simulink model "system_model"  (R2024b)
settings: Solver=ode4  StartTime=0.0  StopTime=T_stop  FixedStep=0.1  RelTol=1e-3
undefined symbols (not defined in the file): bms, dt, SoC_init, T_cool_init, V_RC1_init, V_RC2_init
libraries: simulink x2
settings Model: DataDictionary=buses.sldd  SimulationMode=accelerator  Creator=rayen  LastModifiedBy=rayen
settings OptimizationCC: ZeroExternalMemoryAtStartup=off  ZeroInternalMemoryAtStartup=off
settings DebuggingCC: AlgebraicLoopMsg=error
settings SFSimCC: SimTargetLang=C++
settings RTWCC: TargetLang=C++
settings GRTTargetCC: TargetLangStandard=C++11 (ISO)  CodeInterfacePackaging=C++ class

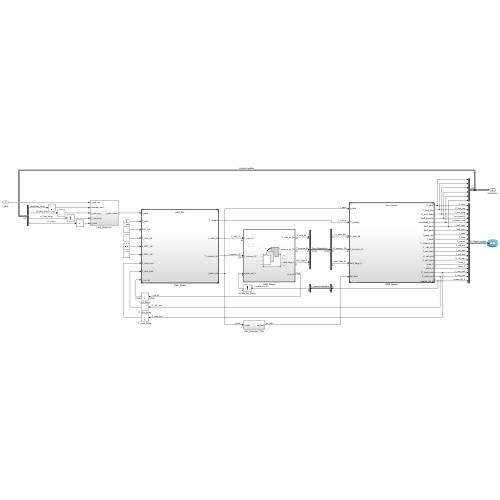
[thumbnail: Simulink's stored preview of the top-level diagram]
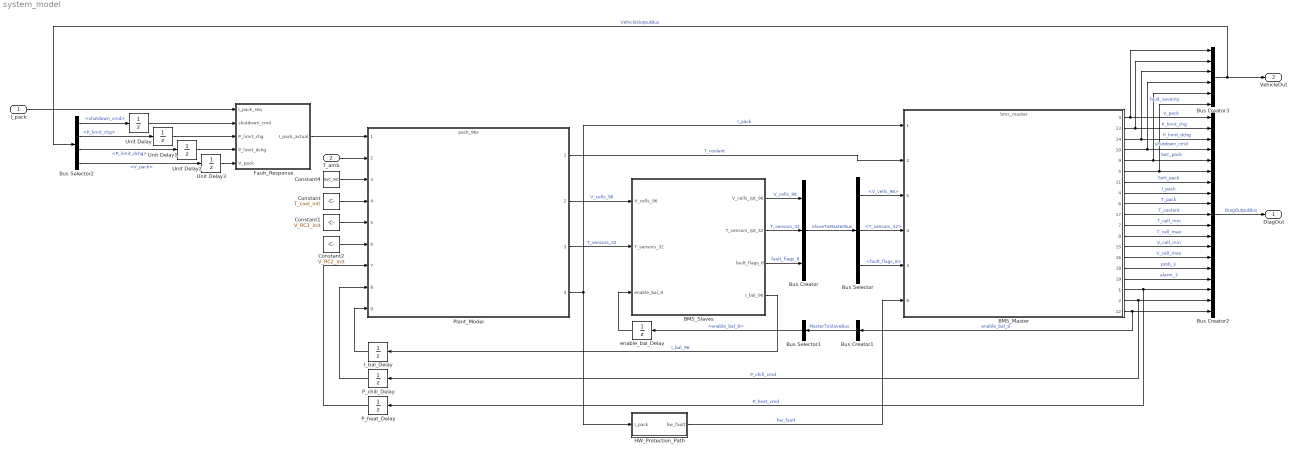
== system system_model ==
  I_pack : Inport  OutDataTypeStr=double
  T_amb : Inport  Port=2  OutDataTypeStr=double
  BMS_Master : ModelReference  ModelNameDialog=bms_master  SimulationMode=Normal  ModelReferenceVersion=1.251
      settings: PortSchema="{\"entries\":[{\"content\":{\"sides\":[{\"content\":{\"connectorIds\":[\"In1\",\"In2\",\"In5\",\"In4\",\"In3\",\"In6\"]},\"type\":\"ConnectorPlacement.EquallySpacedRectSide\",\"uuid\":\"8066489d-2b28-420f-9202-9cd6ff178a29\"},{\"content\":{\"connectorIds\":[\"Out3\",\"Out13\",\"Out14\",\"Out10\",\"Out9\",\"Out5\",\"Out11\",\"Out4\",\"Out6\",\"Out17\",\"Out7\",\"Out8\",\"Out15\",\"Out16\",\"Out18\",\"Out19\",\"Out1\",\"Out2\",\"Out12\"],\"side\":\"RIGHT\"},\"type\":\"ConnectorPlacement.EquallySpacedRectSide\",\"uuid\":\"b076ecb5-2558-4b32-94db-f7a524b49e8a\"},{\"content\":{\"side\":\"TOP\"},\"type\":\"ConnectorPlacement.EquallySpacedRectSide\",\"uuid\":\"5bce71a0-8ae7-4a96-a6b6-c7adac2010e7\"}]},\"type\":\"ConnectorPlacement.EquallySpacedConnector\",\"uuid\":\"27e9bc73-c1a9-451e-b2df-2718d4e67b4c\"}],\"packageUris\":[\"http://schema.mathworks.com/mf0/Connector/R2020b\"],\"version\":\"1.0\"}"
  BMS_Slaves : Subsystem  TreatAsAtomicUnit=on
  Bus Creator : BusCreator  Inputs=3  OutDataTypeStr=Bus: SlaveToMasterBus
  Bus Creator1 : BusCreator  Inputs=1  OutDataTypeStr=Bus: MasterToSlaveBus
  Bus Creator2 : BusCreator  Inputs=19  OutDataTypeStr=Bus: DiagOutputBus
  Bus Creator3 : BusCreator  Inputs=6  OutDataTypeStr=Bus: VehicleOutputBus
  Bus Selector : BusSelector  OutputSignals=V_cells_96,T_sensors_32,fault_flags_8
  Bus Selector1 : BusSelector  OutputSignals=enable_bal_8
  Bus Selector2 : BusSelector  OutputSignals=shutdown_cmd,P_limit_chg,P_limit_dchg,V_pack
  Constant : Constant  Value=T_cool_init
  Constant1 : Constant  Value=V_RC1_init
  Constant2 : Constant  Value=V_RC2_init
  Constant4 : Constant  Value=SoC_init
  Fault_Response : Subsystem
  HW_Protection_Path : Subsystem
  I_bal_Delay : UnitDelay  InitialCondition=zeros(12,8)  SampleTime=dt  HasFrameUpgradeWarning=on
  P_chill_Delay : UnitDelay  SampleTime=dt  HasFrameUpgradeWarning=on
  P_heat_Delay : UnitDelay  SampleTime=dt  HasFrameUpgradeWarning=on
  Plant_Model : ModelReference  ModelNameDialog=pack_96s.slx  SimulationMode=Normal  ModelReferenceVersion=1.65
  Unit Delay : UnitDelay  SampleTime=dt  HasFrameUpgradeWarning=on
  Unit Delay1 : UnitDelay  InitialCondition=96*4.2*150  SampleTime=dt  HasFrameUpgradeWarning=on
  Unit Delay2 : UnitDelay  InitialCondition=96*2.5*405  SampleTime=dt  HasFrameUpgradeWarning=on
  Unit Delay3 : UnitDelay  InitialCondition=96*3.7  SampleTime=dt  HasFrameUpgradeWarning=on
  enable_bal_Delay : UnitDelay  InitialCondition=zeros(1,8)  SampleTime=dt  HasFrameUpgradeWarning=on
  DiagOut : Outport  OutDataTypeStr=Bus: DiagOutputBus
  VehicleOut : Outport  Port=2  OutDataTypeStr=Bus: VehicleOutputBus
  wires:
  T_amb/1 -> Plant_Model/2
  Constant/1 -> Plant_Model/4
  Constant2/1 -> Plant_Model/6
  Constant4/1 -> Plant_Model/3
  Constant1/1 -> Plant_Model/5
  P_heat_Delay/1 -> Plant_Model/7
  Plant_Model/1 -> BMS_Master/2  "T_coolant"
  enable_bal_Delay/1 -> BMS_Slaves/3(enable_bal_8)
  BMS_Slaves/4(I_bal_96) -> I_bal_Delay/1  "I_bal_96"
  I_bal_Delay/1 -> Plant_Model/9
  P_chill_Delay/1 -> Plant_Model/8
  BMS_Slaves/3(fault_flags_8) -> Bus Creator/3  "fault_flags_8"
  BMS_Slaves/2(T_sensors_rpt_32) -> Bus Creator/2  "T_sensors_32"
  BMS_Slaves/1(V_cells_rpt_96) -> Bus Creator/1  "V_cells_96"
  Bus Creator/1 -> Bus Selector/1  "SlaveToMasterBus"
  Bus Creator1/1 -> Bus Selector1/1  "MasterToSlaveBus"
  Bus Selector1/1 -> enable_bal_Delay/1  "<enable_bal_8>"
  Fault_Response/1(I_pack_actual) -> Plant_Model/1
  I_pack/1 -> Fault_Response/1(I_pack_req)
  Unit Delay2/1 -> Fault_Response/4(P_limit_dchg)
  Bus Selector2/2 -> Unit Delay1/1  "<P_limit_chg>"
  Unit Delay3/1 -> Fault_Response/5(V_pack)
  Bus Selector2/4 -> Unit Delay3/1  "<V_pack>"
  Unit Delay1/1 -> Fault_Response/3(P_limit_chg)
  Unit Delay/1 -> Fault_Response/2(shutdown_cmd)
  Bus Selector2/1 -> Unit Delay/1  "<shutdown_cmd>"
  Bus Selector2/3 -> Unit Delay2/1  "<P_limit_dchg>"
  Plant_Model/4 -> HW_Protection_Path/1(I_pack), BMS_Master/1  "I_pack"
  Plant_Model/2 -> BMS_Slaves/1(V_cells_96)  "V_cells_96"
  Plant_Model/3 -> BMS_Slaves/2(T_sensors_32)  "T_sensors_32"
  BMS_Master/3 -> Bus Creator3/1, Bus Creator2/1  "V_pack"
  BMS_Master/13 -> Bus Creator3/2, Bus Creator2/2  "P_limit_chg"
  BMS_Master/14 -> Bus Creator3/3, Bus Creator2/3  "P_limit_dchg"
  BMS_Master/10 -> Bus Creator3/4, Bus Creator2/4  "fault_severity"
  BMS_Master/9 -> Bus Creator3/5, Bus Creator2/5  "shutdown_cmd"
  BMS_Master/5 -> Bus Creator3/6, Bus Creator2/6  "SoC_pack"
  BMS_Master/11 -> Bus Creator2/7  "SoH_pack"
  BMS_Master/4 -> Bus Creator2/8  "I_pack"
  BMS_Master/6 -> Bus Creator2/9  "T_pack"
  BMS_Master/17 -> Bus Creator2/10  "T_coolant"
  BMS_Master/7 -> Bus Creator2/11  "T_cell_min"
  BMS_Master/8 -> Bus Creator2/12  "T_cell_max"
  BMS_Master/15 -> Bus Creator2/13  "V_cell_min"
  BMS_Master/16 -> Bus Creator2/14  "V_cell_max"
  Bus Creator2/1 -> DiagOut/1  "DiagOutputBus"
  Bus Creator3/1 -> VehicleOut/1, Bus Selector2/1  "VehicleOutputBus"
  Bus Selector/1 -> BMS_Master/5  "<V_cells_96>"
  Bus Selector/2 -> BMS_Master/4  "<T_sensors_32>"
  Bus Selector/3 -> BMS_Master/3  "<fault_flags_8>"
  BMS_Master/18 -> Bus Creator2/15  "prob_3"
  BMS_Master/19 -> Bus Creator2/16  "alarm_3"
  BMS_Master/1 -> Bus Creator2/17, P_heat_Delay/1  "P_heat_cmd"
  BMS_Master/2 -> Bus Creator2/18, P_chill_Delay/1  "P_chill_cmd"
  BMS_Master/12 -> Bus Creator1/1, Bus Creator2/19  "enable_bal_8"
  HW_Protection_Path/1(hw_fault) -> BMS_Master/6  "hw_fault"

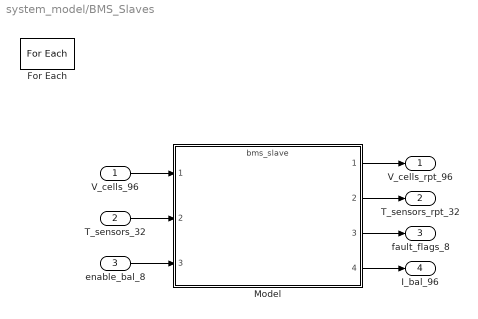
== system system_model/BMS_Slaves ==
  V_cells_96 : Inport  Partition=on  PartitionDimension=1  PartitionWidth=12  PartitionOffset=0
  T_sensors_32 : Inport  Port=2  Partition=on  PartitionDimension=1  PartitionWidth=4  PartitionOffset=0
  enable_bal_8 : Inport  Port=3  Partition=on  PartitionDimension=1  PartitionWidth=1  PartitionOffset=0
  For Each : ForEach  DisableCoverage=on
  Model : ModelReference  ModelNameDialog=bms_slave.slx  ModelReferenceVersion=1.60
  V_cells_rpt_96 : Outport  ConcatenationDimension=1
  T_sensors_rpt_32 : Outport  Port=2  ConcatenationDimension=1
  fault_flags_8 : Outport  Port=3  ConcatenationDimension=1
  I_bal_96 : Outport  Port=4  ConcatenationDimension=2
  wires:
  V_cells_96/1 -> Model/1
  T_sensors_32/1 -> Model/2
  enable_bal_8/1 -> Model/3
  Model/1 -> V_cells_rpt_96/1
  Model/2 -> T_sensors_rpt_32/1
  Model/3 -> fault_flags_8/1
  Model/4 -> I_bal_96/1

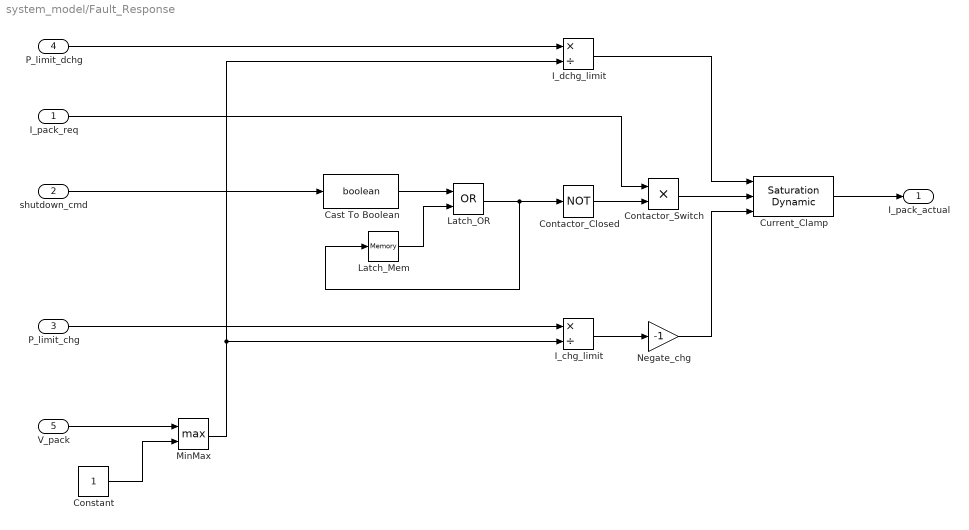
== system system_model/Fault_Response ==
  I_pack_req : Inport
  shutdown_cmd : Inport  Port=2
  P_limit_chg : Inport  Port=3
  P_limit_dchg : Inport  Port=4
  V_pack : Inport  Port=5
  Cast To Boolean : DataTypeConversion  OutDataTypeStr=boolean  SaturateOnIntegerOverflow=off  RndMeth=Floor
  Constant : Constant
  Contactor_Closed : Logic  Operator=NOT  AllPortsSameDT=off  OutDataTypeStr=boolean
  Contactor_Switch : Product
  Current_Clamp : simulink/Discontinuities/Saturation Dynamic  OutMin=[]  OutMax=[]  OutDataTypeStr=Inherit: Same as second input  OutDataType=fixdt(1, 16)  OutScaling=2^-10  DoSatur=off
  I_chg_limit : Product  Inputs=*/
  I_dchg_limit : Product  Inputs=*/
  Latch_Mem : Memory
  Latch_OR : Logic  Operator=OR  AllPortsSameDT=off  OutDataTypeStr=boolean
  MinMax : MinMax  Function=max  Inputs=2
  Negate_chg : Gain  Gain=-1
  I_pack_actual : Outport
  wires:
  Latch_Mem/1 -> Latch_OR/2
  Latch_OR/1 -> Latch_Mem/1, Contactor_Closed/1
  Contactor_Closed/1 -> Contactor_Switch/2
  I_pack_req/1 -> Contactor_Switch/1
  P_limit_chg/1 -> I_chg_limit/1
  V_pack/1 -> MinMax/1
  I_chg_limit/1 -> Negate_chg/1
  P_limit_dchg/1 -> I_dchg_limit/1
  Contactor_Switch/1 -> Current_Clamp/2
  I_dchg_limit/1 -> Current_Clamp/1
  Negate_chg/1 -> Current_Clamp/3
  Current_Clamp/1 -> I_pack_actual/1
  Constant/1 -> MinMax/2
  MinMax/1 -> I_chg_limit/2, I_dchg_limit/2
  Cast To Boolean/1 -> Latch_OR/1
  shutdown_cmd/1 -> Cast To Boolean/1

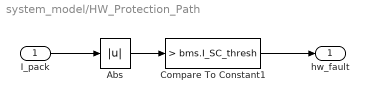
== system system_model/HW_Protection_Path ==
  I_pack : Inport
  Abs : Abs  SaturateOnIntegerOverflow=off
  Compare To Constant1 : simulink/Logic and Bit Operations/Compare To Constant  relop=>  const=bms.I_SC_thresh  OutDataTypeStr=boolean
  hw_fault : Outport
  wires:
  I_pack/1 -> Abs/1
  Abs/1 -> Compare To Constant1/1
  Compare To Constant1/1 -> hw_fault/1
